simulink model "model_1"  (R2022a)
settings: Solver=FixedStepAuto  StartTime=0.0  StopTime=10  FixedStep=0.00001  RelTol=1e-3
values from neighbouring files (symbols this model uses):
  A = [-1, 0, 0, 0 ... (first row only)    [task_1.m]    (also in task_2.m; task_3.m = [0, 3, 0, 0; -3, 0,  0, 0; 0, 0, 0, 1; 0, 0, -1, 0]; task_4.m = [3, -11, -7, 5; -11, 3, -5, 7; -7, -5, 3, 11; 5, 7, 11, 3]; task_4ora.m = [5, -9, -7, 1; -9, 5,  -1, 7; -7, -1, 5, 9; 1, 7, 9, 5])
  B = [0; 5; 0; 6]    [task_1.m]    (also in task_2.m; task_3.m = [0; 0; 0; 0]; task_4.m = [2; 4; 2; 4]; task_4ora.m = [3; 3; 1; 3])
  C = [1, 0, 0, 0; 0, 1, 0, 0; 0, 0, 1, 0; 0, 0, 0, 1]    [task_1.m]    (also in task_2.m; task_3.m = [2, 0, 0, 3]; task_4.m = [2, -2, 2, 2; 2, 4, -2, 4]; task_4ora.m = [2, -2, 2, 2; -2, 4, 2, 4])
  D = zeros(4, 1)    [task_1.m]    (also in task_2.m; task_3.m = 0; task_4.m = 0; task_4ora.m = 0)
  K_1 = Y*inv(P)    [task_1.m]    (also in task_2.m)
  K_2 = Y*inv(P)    [task_1.m]    (also in task_2.m)
  K_3 = Y*inv(P)    [task_1.m]    (also in task_2.m)
  x0 = [-7; -5; 2; 10]    [task_1.m]    (also in task_2.m; task_3.m = [5; -10; 2; -6]; task_4.m = [10; -15; 1; -5]; task_4ora.m = [10; -15; 1; -5])
settings Model: Creator=Family  LastModifiedBy=Family

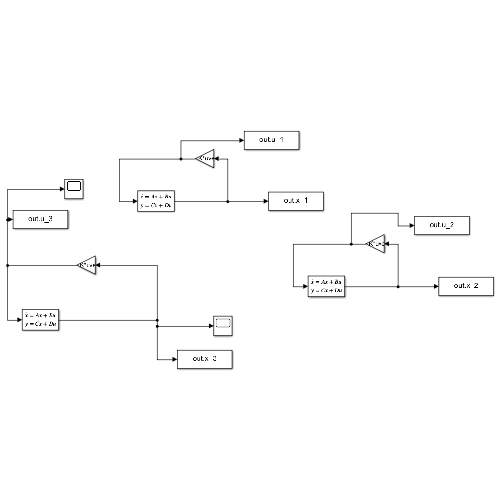
[thumbnail: Simulink's stored preview of the top-level diagram]
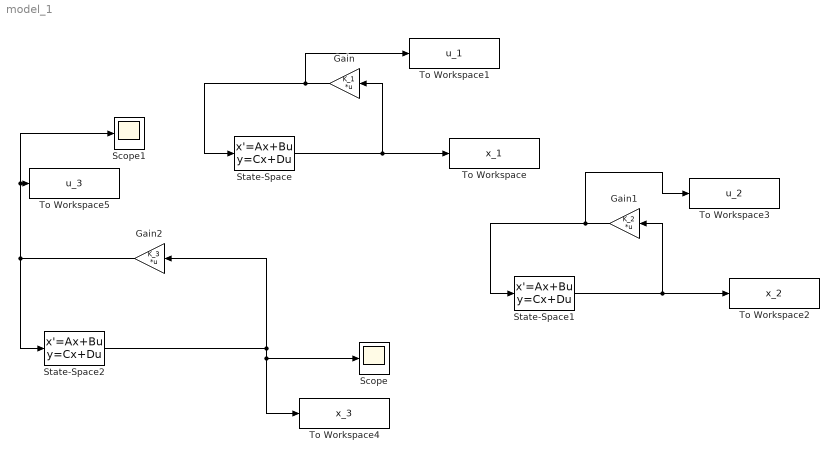
== system model_1 ==
  Gain : Gain  Gain=K_1  Multiplication=Matrix(K*u) (u vector)
  Gain1 : Gain  Gain=K_2  Multiplication=Matrix(K*u) (u vector)
  Gain2 : Gain  Gain=K_3  Multiplication=Matrix(K*u) (u vector)
  Scope : Scope
  Scope1 : Scope
  State-Space : StateSpace  A=A  B=B  C=C  D=D  InitialCondition=x0  ParameterTunability=Unconstrained
  State-Space1 : StateSpace  A=A  B=B  C=C  D=D  InitialCondition=x0  ParameterTunability=Unconstrained
  State-Space2 : StateSpace  A=A  B=B  C=C  D=D  InitialCondition=x0  ParameterTunability=Unconstrained
  To Workspace : ToWorkspace  VariableName=x_1  SaveFormat=Timeseries  SampleTime=-1
  To Workspace1 : ToWorkspace  VariableName=u_1  SaveFormat=Timeseries  SampleTime=0.00001
  To Workspace2 : ToWorkspace  VariableName=x_2  SaveFormat=Timeseries  SampleTime=-1
  To Workspace3 : ToWorkspace  VariableName=u_2  SaveFormat=Timeseries  SampleTime=0.00001
  To Workspace4 : ToWorkspace  VariableName=x_3  SaveFormat=Timeseries  SampleTime=-1
  To Workspace5 : ToWorkspace  VariableName=u_3  SaveFormat=Timeseries  SampleTime=0.00001
  wires:
  Gain2/1 -> Scope1/1, To Workspace5/1, State-Space2/1
  State-Space/1 -> Gain/1, To Workspace/1
  State-Space2/1 -> Scope/1, To Workspace4/1, Gain2/1
  Gain/1 -> To Workspace1/1, State-Space/1
  Gain1/1 -> To Workspace3/1, State-Space1/1
  State-Space1/1 -> Gain1/1, To Workspace2/1
